simulink model "uuvSim_mpc_3dof"  (R2017b)
settings: Solver=ode4  StartTime=0.0  StopTime=10.0  FixedStep=mdl.tStep  RelTol=1e-3
values from neighbouring files (symbols this model uses):
  dt = block.DialogPrm(4).Data    [trj_gen_mpc.m]    (also in trj_gen_mpc_1dof.m; trj_gen_mpc_3dof.m; uuvSimRun_mpc_1dof.m = 0.1; uuvSimRun_mpc_3dof.m = 0.1)
  ics = zeros(12,1)    [uuvSimRun_mpc_1dof.m]    (also in uuvSimRun_mpc_3dof.m)
  p = block.DialogPrm(5).Data    [trj_gen_mpc.m]    (also in trj_gen_mpc_1dof.m; trj_gen_mpc_3dof.m; uuvSimRun_mpc_1dof.m = 25; uuvSimRun_mpc_3dof.m = 25)
  Tinv = pinv(T)    [uuvSimRun_mpc_1dof.m]    (also in uuvSimRun_mpc_3dof.m)
  trj_type = block.DialogPrm(1).Data    [trj_gen_mpc.m]    (also in trj_gen_mpc_1dof.m; trj_gen_mpc_3dof.m; uuvSimRun_mpc_1dof.m = 'minimum_snap'; uuvSimRun_mpc_3dof.m = 'minimum_snap')
  v_c = [0;0;0;0;0;0]    [uuvSimRun_mpc_1dof.m]    (also in uuvSimRun_mpc_3dof.m)
  waypoints = block.DialogPrm(2).Data    [trj_gen_mpc.m]    (also in trj_gen_mpc_1dof.m; trj_gen_mpc_3dof.m; uuvSimRun_mpc_1dof.m = [0,0,0,0,0,0;              2,2,2,0,0,1]; uuvSimRun_mpc_3dof.m = [0,0,0,0,0,0;              2,2,2,0,0,1])
undefined symbols (not defined in the file or in its folder): rov
libraries: mpclib x1
settings Model: Creator=e_anderlini  LastModifiedBy=e_anderlini
settings CodeAppCC: StateflowObjectComments=on

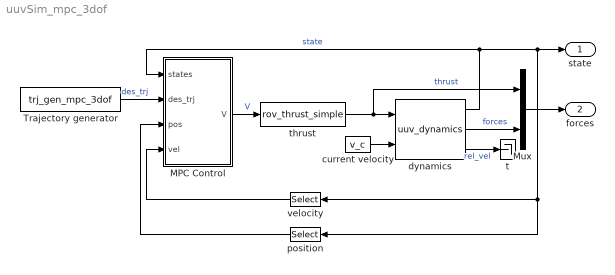
== system uuvSim_mpc_3dof ==
  MPC Control : Subsystem
  Mux : Mux  Inputs=[6,18]
  Trajectory generator : M-S-Function  FunctionName=trj_gen_mpc_3dof  Parameters=trj_type,waypoints,20,dt,p
  current velocity : Constant  Value=v_c
  dynamics : S-Function  FunctionName=uuv_dynamics  Parameters=rov.weight,rov.buoyancy,rov.CoG,rov.CoB,ics,rov.inv_mass',rov.M_A',rov.M_B',rov.D_l',rov.D_q'  SFunctionDeploymentMode=off  EnableBusSupport=off
  position : Selector  InputPortWidth=12  IndexOptions=Index vector (dialog)  Indices=[1 2 3]  OutputSizes=1
  t : Terminator
  thrust : S-Function  FunctionName=rov_thrust_simple  Parameters=rov.coeffs',rov.T'  SFunctionDeploymentMode=off  EnableBusSupport=off
  velocity : Selector  InputPortWidth=12  IndexOptions=Index vector (dialog)  Indices=[7 8 9]  OutputSizes=1
  state : Outport
  forces : Outport  Port=2
  wires:
  dynamics/1 -> velocity/1, position/1, state/1, MPC Control/1("states ")  "state"
  thrust/1 -> Mux/1, dynamics/1  "thrust"
  Mux/1 -> forces/1
  dynamics/2 -> Mux/2  "forces"
  MPC Control/1(V) -> thrust/1  "V"
  dynamics/3 -> t/1  "rel_vel"
  current velocity/1 -> dynamics/2
  position/1 -> MPC Control/3(pos)
  Trajectory generator/1 -> MPC Control/2(des_trj)  "des_trj"
  velocity/1 -> MPC Control/4(vel)

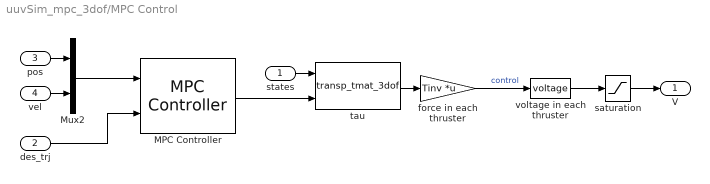
== system uuvSim_mpc_3dof/MPC Control ==
  "states " : Inport
  des_trj : Inport  Port=2
  pos : Inport  Port=3
  vel : Inport  Port=4
  MPC Controller : mpclib/MPC Controller  SCDEnableBlockLinearizationSpecification=on  mpcobj=mpc_kaxan_3dof  is_multiple=0  enable_value=0  return_u0=off  ref_from_ws=off  ref_signal_name=[]  ref_preview=off  md_from_ws=off  md_signal_name=[]  md_preview=off  from_project=off  project_file=MPCtask.mat  md_inport=off  mv_inport=off  cost_outport=off  return_sequence=off  return_qpstatus=off  return_state=off  state_inport=off  lims_inport=off  cc_inport=off  ywt_inport=off  is_designfromscratch=0  uwt_inport=off  duwt_inport=off  rhoeps_inport=off  uref_inport=off  n_ts=0.1  n_p=25  n_mv=3  n_md=0  n_ud=0  n_mo=6  n_uo=0  BlockDataType=double  SampleTimeInherited=off  switch_inport=off
  Mux2 : Mux  Inputs=2
  force in each thruster : Gain  Gain=Tinv  Multiplication=Matrix(K*u)
  saturation : Saturate  UpperLimit=5  LowerLimit=-5
  tau : S-Function  FunctionName=transp_tmat_3dof  SFunctionDeploymentMode=off  EnableBusSupport=off
  voltage in each thruster : S-Function  FunctionName=voltage  Parameters=rov.inv_coeffs'  SFunctionDeploymentMode=off  EnableBusSupport=off
  V : Outport
  wires:
  force in each thruster/1 -> voltage in each thruster/1  "control"
  saturation/1 -> V/1
  MPC Controller/1 -> tau/2
  pos/1 -> Mux2/1
  "states "/1 -> tau/1
  tau/1 -> force in each thruster/1
  voltage in each thruster/1 -> saturation/1
  vel/1 -> Mux2/2
  des_trj/1 -> MPC Controller/2
  Mux2/1 -> MPC Controller/1
